simulink model "slave_robot"  (R2019b)
settings: Solver=VariableStepAuto  StartTime=0.0  StopTime=10.0  RelTol=1e-3
undefined symbols (not defined in the file): Be, Bs, k_s, Kc2v_s, Kd_s, Ke, Kp_s, Ks, Kt2c_s, lArm_s, maxCurrent_s, qe, tau_s
settings Model: Creator=Mirko  LastModifiedBy=Mirko
settings SFSimCC: CustomCodeUndefinedFunction=UseInterfaceOnly

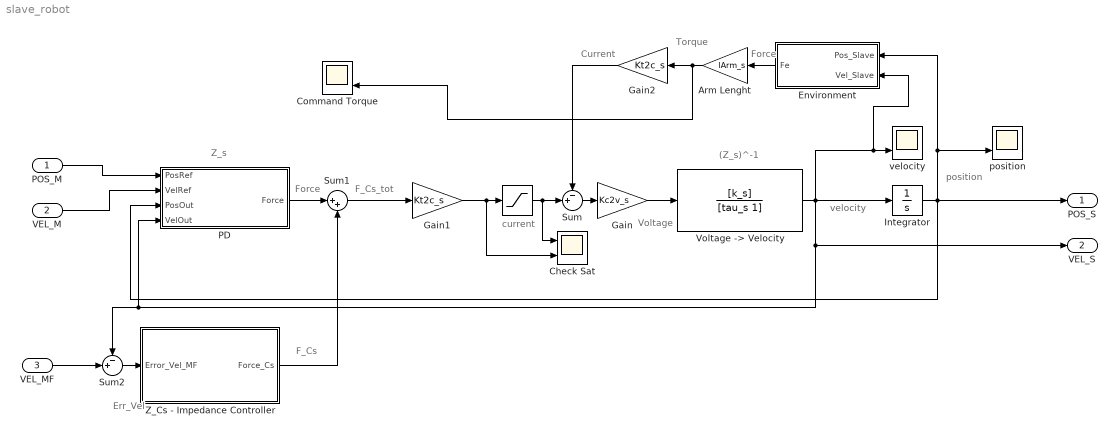
== system slave_robot ==
  note: F_Cs_tot
  note: Err_Vel
  note: F_Cs
  note: Z_s
  note: (Z_s)^-1
  note: Current
  note: Force
  note: Torque
  note: current
  note: Force
  note: Voltage
  note: position
  note: velocity
  "POS_M " : Inport
  VEL_M : Inport  Port=2
  VEL_MF : Inport  Port=3
  " " : Saturate  UpperLimit=maxCurrent_s  LowerLimit=-maxCurrent_s
  Arm Lenght : Gain  Gain=lArm_s
  Check Sat : Scope  NumInputPorts=2
  Command Torque : Scope  NumInputPorts=2
  "Environment " : Subsystem
  Gain : Gain  Gain=Kc2v_s
  Gain1 : Gain  Gain=Kt2c_s
  Gain2 : Gain  Gain=Kt2c_s
  Integrator : Integrator
  PD : Subsystem
  Sum : Sum  Inputs=-+|
  Sum1 : Sum  Inputs=|++
  Sum2 : Sum  Inputs=-+|
  "Voltage -> Velocity " : TransferFcn  Numerator=[k_s]  Denominator=[tau_s 1]
  Z_Cs - Impedance Controller : Subsystem
  position : Scope  NumInputPorts=2
  velocity : Scope  NumInputPorts=2
  POS_S : Outport
  VEL_S : Outport  Port=2
  wires:
  "Voltage -> Velocity "/1 -> Integrator/1, "Environment "/2("Vel_Slave "), velocity/2, VEL_S/1, Sum2/1, PD/4(VelOut)
  Integrator/1 -> "Environment "/1(Pos_Slave), position/2, POS_S/1, PD/3(PosOut)
  " "/1 -> Check Sat/1, Sum/2
  Gain/1 -> "Voltage -> Velocity "/1
  Gain1/1 -> Check Sat/2, " "/1
  "Environment "/1(Fe) -> Arm Lenght/1
  Arm Lenght/1 -> Gain2/1, Command Torque/2
  Sum/1 -> Gain/1
  Gain2/1 -> Sum/1
  VEL_M/1 -> PD/2(VelRef)
  "POS_M "/1 -> PD/1(PosRef)
  VEL_MF/1 -> Sum2/2
  Sum2/1 -> Z_Cs - Impedance Controller/1(Error_Vel_MF)
  PD/1(Force) -> Sum1/1
  Z_Cs - Impedance Controller/1("Force_Cs ") -> Sum1/2
  Sum1/1 -> Gain1/1

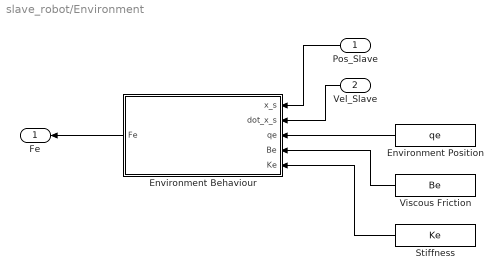
== system slave_robot/Environment  ==
  Pos_Slave : Inport
  "Vel_Slave " : Inport  Port=2
  Environment Behaviour : MATLAB Function  TreatAsAtomicUnit=on
  Environment Position : Constant  Value=qe
  Stiffness : Constant  Value=Ke
  Viscous Friction : Constant  Value=Be
  Fe : Outport
  wires:
  Pos_Slave/1 -> Environment Behaviour/1(x_s)
  "Vel_Slave "/1 -> Environment Behaviour/2(dot_x_s)
  Environment Position/1 -> Environment Behaviour/3(qe)
  Viscous Friction/1 -> Environment Behaviour/4(Be)
  Stiffness/1 -> Environment Behaviour/5(Ke)
  Environment Behaviour/1(Fe) -> Fe/1

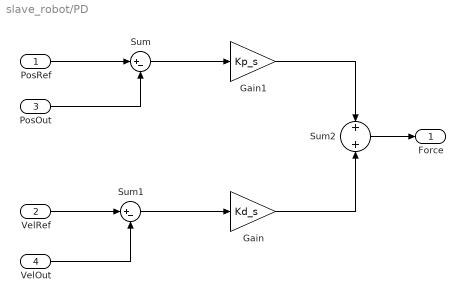
== system slave_robot/PD ==
  PosRef : Inport
  VelRef : Inport  Port=2
  PosOut : Inport  Port=3
  VelOut : Inport  Port=4
  Gain : Gain  Gain=Kd_s
  Gain1 : Gain  Gain=Kp_s
  Sum : Sum  Inputs=|+-
  Sum1 : Sum  Inputs=|+-
  Sum2 : Sum
  Force : Outport
  wires:
  PosRef/1 -> Sum/1
  PosOut/1 -> Sum/2
  VelRef/1 -> Sum1/1
  VelOut/1 -> Sum1/2
  Sum1/1 -> Gain/1
  Sum/1 -> Gain1/1
  Gain1/1 -> Sum2/1
  Gain/1 -> Sum2/2
  Sum2/1 -> Force/1

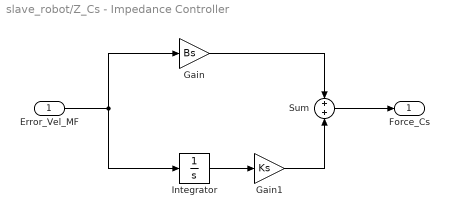
== system slave_robot/Z_Cs - Impedance Controller ==
  Error_Vel_MF : Inport
  Gain : Gain  Gain=Bs
  Gain1 : Gain  Gain=Ks
  Integrator : Integrator
  Sum : Sum
  "Force_Cs " : Outport
  wires:
  Error_Vel_MF/1 -> Gain/1, Integrator/1
  Integrator/1 -> Gain1/1
  Gain/1 -> Sum/1
  Gain1/1 -> Sum/2
  Sum/1 -> "Force_Cs "/1

== matlab function slave_robot/Environment /Environment Behaviour ==
  data: x_s input; Fe output; dot_x_s input; qe input; Be input; Ke input
function Fe = Env(x_s, dot_x_s, qe, Be, Ke)
    
    if(x_s > qe)
        Fe = Ke*(x_s - qe) + Be*dot_x_s;
    else
        Fe = 0;
    end
